simulink model "NL_1DOF"  (R2019b)
settings: Solver=VariableStepAuto  StartTime=0.0  StopTime=50  RelTol=1e-3
InitFcn:
  | load("parameters.mat")
  | load("Coefficients.mat")
undefined symbols (not defined in the file): Dm, Dt, g, Jeq, k_pitch_, Mb, p_sat_Hor_touch, w_ramp_0N, w_ramp_0P, w_ramp_1N, w_ramp_1P
settings Model: Creator=peter  LastModifiedBy=lbend

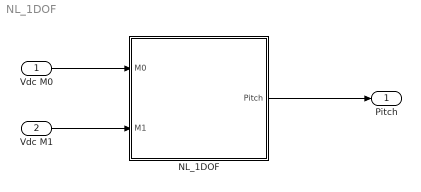
== system NL_1DOF ==
  Vdc M0 : Inport
  Vdc M1 : Inport  Port=2
  NL_1DOF : Subsystem
      mask Display: image('C:\Users\lbend\OneDrive - Politecnico di Milano\Root Locos\Reports\Photos&Images\1doF.png'); % Use "Edit Image" on toolstrip to change.
  Pitch : Outport
  wires:
  Vdc M0/1 -> NL_1DOF/1(M0)
  Vdc M1/1 -> NL_1DOF/2("M1 ")
  NL_1DOF/1(Pitch) -> Pitch/1

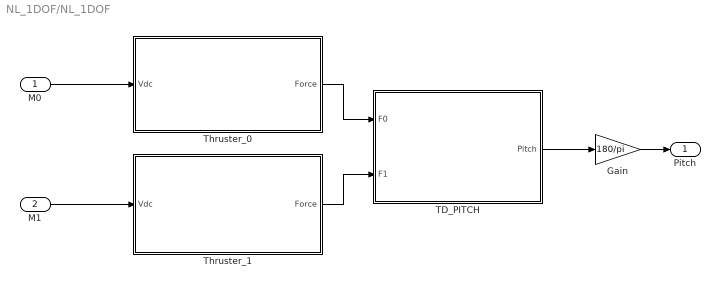
== system NL_1DOF/NL_1DOF ==
  M0 : Inport
  "M1 " : Inport  Port=2
  Gain : Gain  Gain=180/pi
  TD_PITCH : Subsystem
  Thruster_0 : Subsystem
  "Thruster_1 " : Subsystem
  Pitch : Outport
  wires:
  M0/1 -> Thruster_0/1(Vdc)
  "M1 "/1 -> "Thruster_1 "/1(Vdc)
  TD_PITCH/1(Pitch) -> Gain/1
  Thruster_0/1(Force) -> TD_PITCH/1(F0)
  "Thruster_1 "/1(Force) -> TD_PITCH/2("F1 ")
  Gain/1 -> Pitch/1

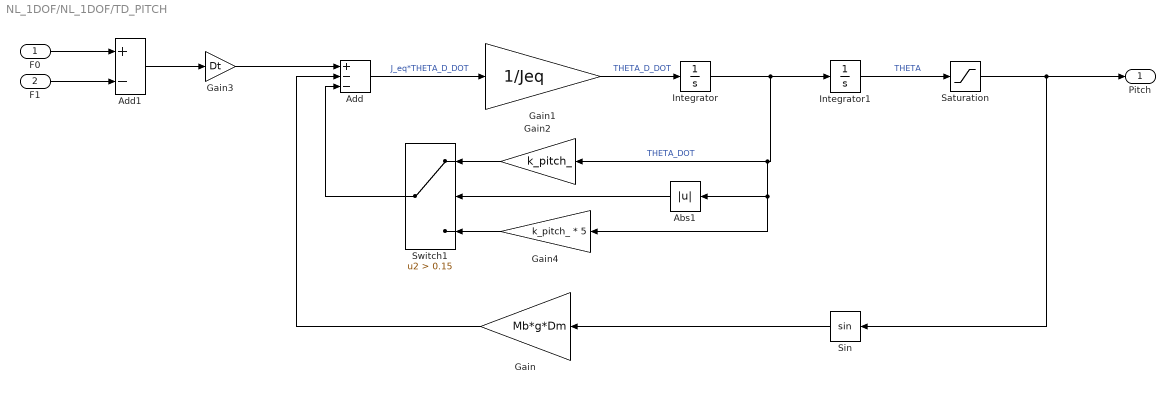
== system NL_1DOF/NL_1DOF/TD_PITCH ==
  F0 : Inport
  "F1 " : Inport  Port=2
  Abs1 : Abs
  Add : Sum  Inputs=+--
  Add1 : Sum  Inputs=+-
  Gain : Gain  Gain=Mb*g*Dm
  Gain1 : Gain  Gain=1/Jeq
  Gain2 : Gain  Gain=k_pitch_
  Gain3 : Gain  Gain=Dt
  Gain4 : Gain  Gain=k_pitch_ * 5
  Integrator : Integrator
  Integrator1 : Integrator
  Saturation : Saturate  UpperLimit=p_sat_Hor_touch  LowerLimit=-p_sat_Hor_touch
  Sin : Trigonometry
  Switch1 : Switch  Criteria=u2 > Threshold  Threshold=0.15
  Pitch : Outport
  wires:
  Integrator/1 -> Gain2/1, Gain4/1, Abs1/1, Integrator1/1  "THETA_DOT"
  Gain3/1 -> Add/1
  "F1 "/1 -> Add1/2
  Add1/1 -> Gain3/1
  Saturation/1 -> Pitch/1, Sin/1
  Gain1/1 -> Integrator/1  "THETA_D_DOT"
  Integrator1/1 -> Saturation/1  "THETA"
  Gain/1 -> Add/2
  Abs1/1 -> Switch1/2
  Switch1/1 -> Add/3
  Sin/1 -> Gain/1
  F0/1 -> Add1/1
  Add/1 -> Gain1/1  "J_eq*THETA_D_DOT"
  Gain4/1 -> Switch1/3
  Gain2/1 -> Switch1/1

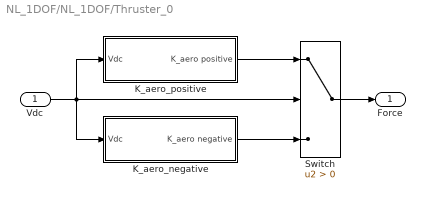
== system NL_1DOF/NL_1DOF/Thruster_0 ==
  Vdc : Inport
  K_aero_negative : Subsystem
  K_aero_positive : Subsystem
  Switch : Switch  Criteria=u2 > Threshold
  Force : Outport
  wires:
  Switch/1 -> Force/1
  K_aero_positive/1(K_aero positive) -> Switch/1
  Vdc/1 -> K_aero_positive/1(Vdc), K_aero_negative/1(Vdc), Switch/2
  K_aero_negative/1(K_aero negative) -> Switch/3

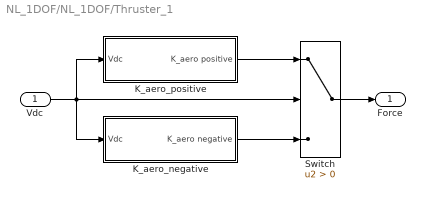
== system NL_1DOF/NL_1DOF/Thruster_1  ==
  Vdc : Inport
  K_aero_negative : Subsystem
  K_aero_positive : Subsystem
  Switch : Switch  Criteria=u2 > Threshold
  Force : Outport
  wires:
  Switch/1 -> Force/1
  K_aero_positive/1(K_aero positive) -> Switch/1
  Vdc/1 -> K_aero_negative/1(Vdc), Switch/2, K_aero_positive/1(Vdc)
  K_aero_negative/1(K_aero negative) -> Switch/3

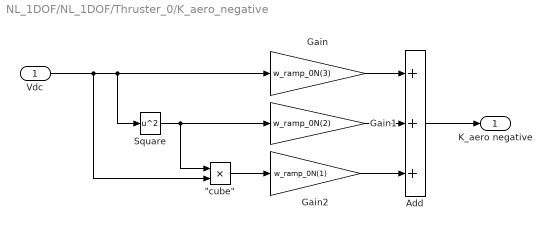
== system NL_1DOF/NL_1DOF/Thruster_0/K_aero_negative ==
  Vdc : Inport
  "\"cube\"" : Product  Inputs=**
  Add : Sum  Inputs=+++
  Gain : Gain  Gain=w_ramp_0N(3)
  Gain1 : Gain  Gain=w_ramp_0N(2)
  Gain2 : Gain  Gain=w_ramp_0N(1)
  Square : Math  Operator=square  SignedPower=off  SaturateOnIntegerOverflow=on
  K_aero negative : Outport
  wires:
  Vdc/1 -> "\"cube\""/2, Square/1, Gain/1
  Gain/1 -> Add/1
  Square/1 -> "\"cube\""/1, Gain1/1
  Gain1/1 -> Add/2
  Gain2/1 -> Add/3
  "\"cube\""/1 -> Gain2/1
  Add/1 -> K_aero negative/1

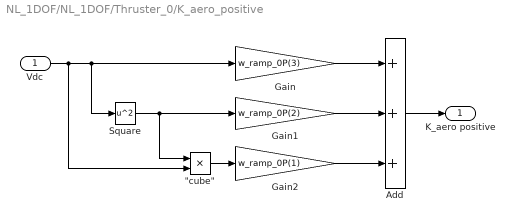
== system NL_1DOF/NL_1DOF/Thruster_0/K_aero_positive ==
  Vdc : Inport
  "\"cube\"" : Product  Inputs=**
  Add : Sum  Inputs=+++
  Gain : Gain  Gain=w_ramp_0P(3)
  Gain1 : Gain  Gain=w_ramp_0P(2)
  Gain2 : Gain  Gain=w_ramp_0P(1)
  Square : Math  Operator=square  SignedPower=off  SaturateOnIntegerOverflow=on
  K_aero positive : Outport
  wires:
  Vdc/1 -> Gain/1, Square/1, "\"cube\""/2
  Add/1 -> K_aero positive/1
  Gain/1 -> Add/1
  Square/1 -> "\"cube\""/1, Gain1/1
  Gain1/1 -> Add/2
  "\"cube\""/1 -> Gain2/1
  Gain2/1 -> Add/3

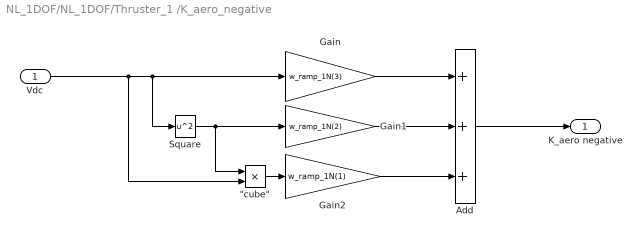
== system NL_1DOF/NL_1DOF/Thruster_1 /K_aero_negative ==
  Vdc : Inport
  "\"cube\"" : Product  Inputs=**
  Add : Sum  Inputs=+++
  Gain : Gain  Gain=w_ramp_1N(3)
  Gain1 : Gain  Gain=w_ramp_1N(2)
  Gain2 : Gain  Gain=w_ramp_1N(1)
  Square : Math  Operator=square  SignedPower=off  SaturateOnIntegerOverflow=on
  K_aero negative : Outport
  wires:
  Vdc/1 -> "\"cube\""/2, Square/1, Gain/1
  Gain/1 -> Add/1
  Square/1 -> "\"cube\""/1, Gain1/1
  Gain1/1 -> Add/2
  Gain2/1 -> Add/3
  "\"cube\""/1 -> Gain2/1
  Add/1 -> K_aero negative/1

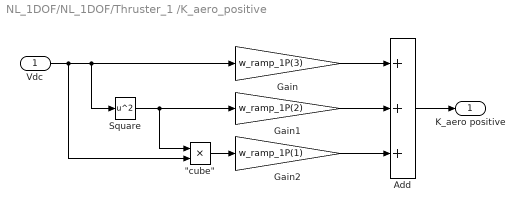
== system NL_1DOF/NL_1DOF/Thruster_1 /K_aero_positive ==
  Vdc : Inport
  "\"cube\"" : Product  Inputs=**
  Add : Sum  Inputs=+++
  Gain : Gain  Gain=w_ramp_1P(3)
  Gain1 : Gain  Gain=w_ramp_1P(2)
  Gain2 : Gain  Gain=w_ramp_1P(1)
  Square : Math  Operator=square  SignedPower=off  SaturateOnIntegerOverflow=on
  K_aero positive : Outport
  wires:
  Vdc/1 -> Gain/1, Square/1, "\"cube\""/2
  Add/1 -> K_aero positive/1
  Gain/1 -> Add/1
  Square/1 -> "\"cube\""/1, Gain1/1
  Gain1/1 -> Add/2
  "\"cube\""/1 -> Gain2/1
  Gain2/1 -> Add/3
